simulink model "sim_test"  (R2013b)
settings: Solver=ode45  StartTime=0.0  StopTime=10.0  RelTol=1e-3
settings Model: Creator=tonegas  LastModifiedBy=tonegas

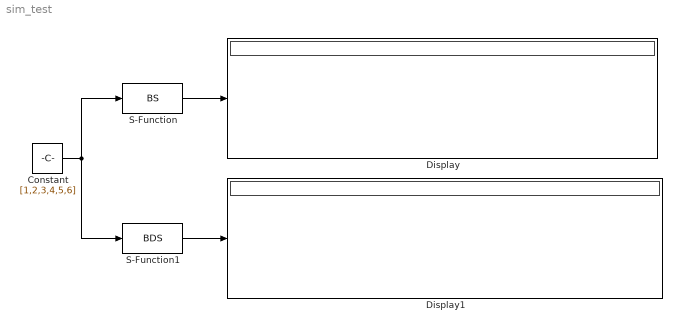
== system sim_test ==
  Constant : Constant  Value=[1,2,3,4,5,6]
  Display : Display
  Display1 : Display
  S-Function : S-Function  FunctionName=BS  EnableBusSupport=off
  S-Function1 : S-Function  FunctionName=BDS  EnableBusSupport=off
  wires:
  Constant/1 -> S-Function/1, S-Function1/1
  S-Function/1 -> Display/1
  S-Function1/1 -> Display1/1
